simulink model "Copy_of_indy7_dualArm"  (R2024b)
settings: Solver=FixedStepAuto  StartTime=0.0  StopTime=10  FixedStep=0.001  RelTol=1e-3
model workspace (MAT data in the model file):
  joint_friction = [80 80 20 10 10 5]
  lambda_l_list = [0 -1.17357539658 0.993815552956 -2.091 0 0 -0.111945470246 0.0246912114191 0.243747835972 1.20917417944 1.20917417944 -1.20905770917 ... (42 elements, 6x7)]
  lambda_r_list = [0 1.17618914658 0.992300581915 2.091 0 0 -0.111945470246 0.0246912114191 0.243747835972 1.20917417944 1.20917417944 -1.20905770917 ... (42 elements, 6x7)]
  lambda_rl_list = [2.58853268681e-20 -2.25514051877e-16 -0.06 -1.83339582048e-16 -4.06575814682e-20 0 0.0911029490978 -0.02862210596 -0.174516399919 1.20917417944 1.20905770917 -1.20917417944 ... (78 elements, 6x13)]
  q_init_l : Simulink.Parameter (value not decoded)
  q_init_l1 : Simulink.Parameter (value not decoded)
  q_init_l2 : Simulink.Parameter (value not decoded)
  q_init_l3 : Simulink.Parameter (value not decoded)
  q_init_l4 : Simulink.Parameter (value not decoded)
  q_init_l5 : Simulink.Parameter (value not decoded)
  q_init_l6 : Simulink.Parameter (value not decoded)
  q_init_r : Simulink.Parameter (value not decoded)
  q_init_r1 : Simulink.Parameter (value not decoded)
  q_init_r2 : Simulink.Parameter (value not decoded)
  q_init_r3 : Simulink.Parameter (value not decoded)
  q_init_r4 : Simulink.Parameter (value not decoded)
  q_init_r5 : Simulink.Parameter (value not decoded)
  q_init_r6 : Simulink.Parameter (value not decoded)
  robot : robotics.RigidBodyTree (value not decoded)
values from neighbouring files (symbols this model uses):
  lambda_lr_list = [lambda_lr_list,-lambda_rl_list(:,i)]    [getDualArmLambdaList.m]    (also in untitled3.m)
  m = models{k}    [code_generation.m]
  N = length(q)    [FKLocalPOE.m]
symbols that are objects in the model workspace (value not decoded): q_init_l, q_init_l1, q_init_r
undefined symbols (not defined in the file or in its folder): Blist_tcp, DiscIntNeverNeededParam, dt, exp6, M_tcp, q_init, q_max, q_min, qdot_max, qdot_min, SW_a, SW_b0, X, Y, Z
libraries: sm_lib x148, nesl_utility x45, robotmaniplib x9, robotcorelib x5, simulink x4, matrix_library x2
(part 5 of 5)

== matlab function Copy_of_indy7_dualArm/DualArmTaskSpaceController/SPDControllerWithQP_Right1 ==
  data: M input; cvec input; q input size=[12,1]; qddot output size=[6,1]; qdot input size=[12,1]; Tdes input size=[4,4]; Vdes input size=[6,1]; Vdotdes input size=[6,1]; T input size=[4,4]; V input size=[6,1]; J input size=[6,6]; Jdot input size=[6,6]; qinit input size=[6,1]; qdot_max input size=[6,1]; qdot_min input size=[6,1]; q_max input size=[6,1]; q_min input size=[6,1]; TaskKp input size=[1,6]; TaskKv input size=[1,6]; dt input; a input; b0 input
function qddot = SPDImplicitEuler(M,cvec,q,qdot,Tdes,Vdes,Vdotdes,T,V,J,Jdot,qinit,qdot_max,qdot_min,q_max,q_min,TaskKp,TaskKv,dt,a,b0)
    % Tdes(2,4) = Tdes(2,4)+0.3*sin(2*pi*t/5);
    M = M(7:end,7:end);
    qdot  = qdot(7:end);
    q = q(7:end);
    cvec = cvec(7:end);

    % % Tdes(3,4) = Tdes(3,4)+0.5*sin(2*pi*t/5);

    TaskKp = diag(TaskKp);
    TaskKv = diag(TaskKv);


    Ttilde = TransInv(T)*Tdes;
    lambda  = log6(Ttilde);
    Vtilde = Vdes-Adjoint(TransInv(Ttilde))*V;
    dlambda = dexp6(-lambda)*Vtilde;
    AdInvT = Adjoint(TransInv(Ttilde));
    D = dlog6(-lambda)*Vdotdes-dlog6(-lambda)*AdInvT*Jdot*qdot+dlog6(-lambda)*ad(Vtilde)*Vdes-dlog6(-lambda)*ddexp6(-lambda,-dlambda)*dlambda;
    % qddot = (M+JT*TaskKv*dt*dlog6(-lambda)*AdInvT*J)\(JT*TaskKp*(lambda)+JT*TaskKp*dt*dlambda+JT*TaskKv*dlambda+(eye(7)-pinv(J)*J)*(Kinit*(qinit-q)+Dinit*(-qdot))-B*qdot);
    
    
      
    Jlambda = -dlog6(lambda)*J;
    Vtilde = Adjoint(TransInv(Ttilde))*Vdes-V;
    lambdadot = dlog6(lambda)*Vtilde;
    lambda_next = lambda+lambdadot*dt;
    B = b0 * exp(-det(J)*det(J)/ a / a) * eye(length(q));

    JlambdaT = Jlambda';
    Gamma = dlog6(lambda_next)*Adjoint(exp6(-lambda_next))*(Vdes+dt*Vdotdes)-dlog6(lambda_next)*V-dlog6(lambda_next)*dt*Jdot*qdot;
    qddot = (M+JlambdaT*TaskKv*dt*Jlambda)\(JlambdaT*(-TaskKp*lambda_next-TaskKv*Gamma)-cvec-B*qdot);


    % Js_prime= JacobianSpace(Slist6,q(2:end));
    % Jsdot_prime= dJacobianSpace(Js_prime,qdot(2:end));
    % Tbase_tcp =FKinSpace(M_tcp,Slist6,q(2:end));
    % p = Tbase_tcp(1:3,4);
    % pdot = Js_prime(1:3,:)*qdot(2:end);
    % 
    % 
    % p_max = 2.5;
    % lambda = 0.1;
    % 
    H = eye(6);
    % H = H+lambda*eye(6);

    f = -2*qddot;
    % f = f-lambda*qddot_prev;
    % Ao = Js_prime(1,:)*[zeros(6,1) eye(6)];

    Au = eye(6);
    bu = 10*[qdot_max-qdot];
    bl = -10*[qdot-qdot_min];
    alpha1 = 1;
    alpha3 = 10;
    beta1 = 10;
    beta3 = 100;
    Aq =eye(6);
    bqu = [-(alpha1+alpha3)*qdot+(alpha1*alpha3)*(q_max-q)];
    bql = [-(alpha1+alpha3)*qdot-(alpha1*alpha3)*(q-q_min)];
    % bou = [-(beta1+beta3)*pdot(1)+(beta1*beta3)*(p_max-p(1))-Jsdot_prime(1,:)*qdot(2:end)];

    x0 = qddot;

    A = [Au;-Au;Aq;-Aq];
    b = [bu;-bl;bqu;-bql];
    % A = [Au;-Au;Aq;-Aq];
    % b = [bu;-bl;bqu;-bql];
    options = optimoptions('quadprog', ...
                           'Algorithm','active-set', ...
                           'Display','off');

    % 4) quadprog 호출
    [x, fval, exitflag, output, lambda] = quadprog( ...
        H, f, A, b, [], [], [], [], x0, options);
    if(exitflag>0)
        qddot =x;
    else

    end

== matlab function Copy_of_indy7_dualArm/Kinematics/MATLAB Function1 ==
  data: q input; q_lr output
function q_lr = getQrel(q)
dnfunction q_lr = getQrel(q)
q_lr = zeros(12,1);
q_lr = [-flip(q(1:6));q(7:end)];

== matlab function Copy_of_indy7_dualArm/Kinematics/MATLAB Function ==
  data: Jdot output; J output; lambda_list input; T output; q input; q_dot input
function [Jdot,J,T]=FKJacobian(lambda_list,q,q_dot)
    Ti = eye(4);
    [m,n]=size(lambda_list);
    lamda_z = [0,0,0,0,0,1]';
    ez = [0,0,1]';
    N = length(q);
    J = zeros(6,N);
    Jdot=zeros(6,N);
  
    Ti = exp6(lambda_list(:,end));
    [Ri,pi] = TransToRp(Ti);
    J(:,end)=[Ri'*VecToso3(ez)*pi;Ri'*ez];
    for i =N:-1:1
        Ti = exp6(lambda_list(:,i))*exp6(lamda_z*q(i))*Ti;
 
        [Ri,pi] = TransToRp(Ti);
        if i>1
            J(:,i-1)=[Ri'*VecToso3(ez)*pi;Ri'*ez];
        end

    end
    for i=1:1:N
        Ji = J(:,i);
        dJidt = zeros(6,1);
        for j=1:1:N
            Jj = J(:,j);
            aJiaqj = zeros(6,1);
            if(i<j) 
                aJiaqj = ad(Ji)*Jj;
            end
            dJidt = dJidt+aJiaqj*q_dot(j);
        end
        Jdot(:,i) = dJidt;
    end
    T = Ti;
end

== matlab function Copy_of_indy7_dualArm/Kinematics/MATLAB Function2 ==
  data: q input; q_lr output
function q_lr = getQrel(q)
q_lr = zeros(12,1);
q_lr = [-flip(q(1:6));q(7:end)];

== matlab function Copy_of_indy7_dualArm/DualArm/MATLAB Function ==
  data: R input; T output; p input
function T = RpToTrans(R,p)
 T = RpToTrans(R,p);

== matlab function Copy_of_indy7_dualArm/DualArm/MATLAB Function1 ==
  data: R input; T output; p input
function T = RpToTrans(R,p)
 T = RpToTrans(R,p);

== matlab function Copy_of_indy7_dualArm/DualArm/MATLAB Function2 ==
  data: T_r input; T_rl output; T_l input
function T_rl = fcn(T_r,T_l)

T_rl = TransInv(T_r)*T_l;

== matlab function Copy_of_indy7_dualArm/Kinematics/MATLAB Function7 ==
  data: Jdot output; J output; lambda_list input; T output; q input; q_dot input
function [Jdot,J,T]=FKJacobian(lambda_list,q,q_dot)
    Ti = eye(4);
    [m,n]=size(lambda_list);
    lamda_z = [0,0,0,0,0,1]';
    ez = [0,0,1]';
    N = length(q);
    J = zeros(6,N);
    Jdot=zeros(6,N);
  
    Ti = exp6(lambda_list(:,end));
    [Ri,pi] = TransToRp(Ti);
    J(:,end)=[Ri'*VecToso3(ez)*pi;Ri'*ez];
    for i =N:-1:1
        Ti = exp6(lambda_list(:,i))*exp6(lamda_z*q(i))*Ti;
 
        [Ri,pi] = TransToRp(Ti);
        if i>1
            J(:,i-1)=[Ri'*VecToso3(ez)*pi;Ri'*ez];
        end

    end
    for i=1:1:N
        Ji = J(:,i);
        dJidt = zeros(6,1);
        for j=1:1:N
            Jj = J(:,j);
            aJiaqj = zeros(6,1);
            if(i<j) 
                aJiaqj = ad(Ji)*Jj;
            end
            dJidt = dJidt+aJiaqj*q_dot(j);
        end
        Jdot(:,i) = dJidt;
    end
    T = Ti;
end
